simulink model "RC_circuit"  (R2020b)
settings: Solver=VariableStepAuto  StartTime=0.0  StopTime=10.0  RelTol=1e-3
PreLoadFcn:
  | R =10;
  | c = 10 ;
settings Model: Creator=Admin  LastModifiedBy=Admin

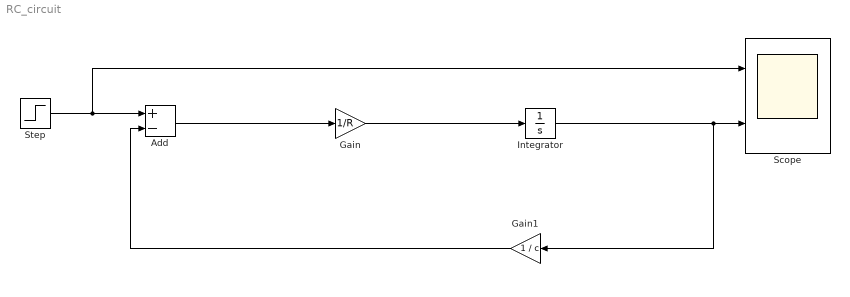
== system RC_circuit ==
  Add : Sum  Inputs=+-
  Gain : Gain  Gain=1/R
  Gain1 : Gain  Gain=1 / c
  Integrator : Integrator
  Scope : Scope  NumInputPorts=2
  Step : Step  SampleTime=0
  wires:
  Gain/1 -> Integrator/1
  Add/1 -> Gain/1
  Gain1/1 -> Add/2
  Step/1 -> Scope/1, Add/1
  Integrator/1 -> Gain1/1, Scope/2
